simulink model "CompFeatures_eqHarness_req"  (R2012b)
settings: Solver=FixedStepDiscrete  StartTime=0.0  StopTime=50  RelTol=1e-3
InitFcn:
  | N=256;
  | Fs = 1000;
  | bw = 5.6;
undefined symbols (not defined in the file): sigbuilder_block
libraries: simulink x1
settings Model: RequirementInfo={'other' '..\..\..\requirements\ebd_srs.doc' '@Simulink_requirement_item_4' 'true' 'Filter input signal via polyphase digital filter bank' 'Requirement' } %GIDa_bfa4a348_cd9f_4101_a776_3ea215f34dae  SldvGeneratedHarnessModel=TestUnitModel=CompFeatures|  CovMetricSettings=dcmoe  CovHTMLOptions=-aTS=1 -bRG=1 -bTC=0 -hTR=0 -nFC=0 -scm=1 -bcm=1  CovModelRefEnable=on  CovExternalEMLEnable=on  Creator=aanantha  LastModifiedBy=klindqvi
settings DataIOCC: SaveFormat=StructureWithTime  SignalLoggingSaveFormat=ModelDataLogs  SaveOutput=off  SaveTime=off  SignalLoggingName=logsOut
settings OptimizationCC: InlineParams=on  OptimizeModelRefInitCode=on  LifeSpan=1
settings DebuggingCC: ReadBeforeWriteMsg=DisableAll  WriteAfterWriteMsg=DisableAll  WriteAfterReadMsg=DisableAll  InheritedTsInSrcMsg=none  ParameterPrecisionLossMsg=none  FcnCallInpInsideContextMsg=EnableAllAsWarning
settings HardwareCC: ProdLargestAtomicInteger=Long  ProdLargestAtomicFloat=Double  ProdEndianess=LittleEndian  ProdHWDeviceType=ARM Compatible->ARM Cortex
settings ModelReferenceCC: CheckModelReferenceTargetMessage=none
settings RTWCC: SystemTargetFile=ert.tlc  GenCodeOnly=on  TemplateMakefile=ert_default_tmf  Description=Embedded Coder  GenerateReport=on  ProcessScript=ert_make_rtw_hook  IncludeHyperlinkInReport=on  LaunchReport=on  GenerateTraceInfo=on  GenerateTraceReportSl=on  GenerateTraceReportSf=on  GenerateTraceReportEml=on  GenerateCodeMetricsReport=on
settings CodeAppCC: IgnoreCustomStorageClasses=off
settings ERTTargetCC: CodeReplacementLibrary=GCC ARM Cortex-A8  MultiwordLength=2048  GenerateSampleERTMain=on  ERTCustomFileTemplate=example_file_process.tlc  ConvertIfToSwitch=off  SuppressUnreachableDefaultCases=off

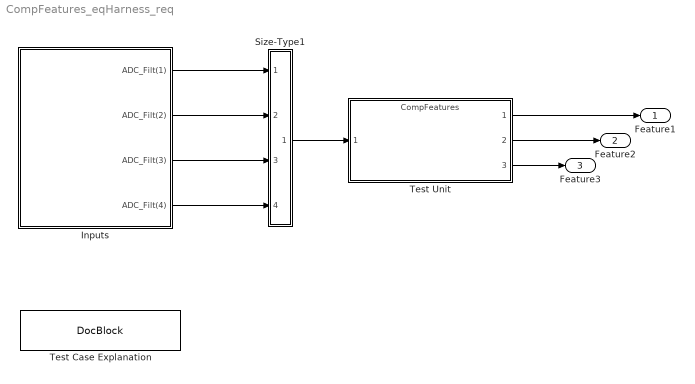
== system CompFeatures_eqHarness_req ==
  Inputs : Subsystem  Tag=STV Subsys  LoadFcn=sigbuilder_block('load',[49.5 50.25 519.75 603 ]);  StartFcn=sigbuilder_block('start');  StopFcn=sigbuilder_block('stop');  ClipboardFcn=sigbuilder_block('clipboard');  mask(Sigbuilder block){}
      mask init:
      | if ~strcmp(get_param(bdroot(gcb),'SimulationStatus'),'stopped'),tuvar = sigbuilder_block('maskInit'); end
      settings: CopyFcn=sigbuilder_block('copy');  DeleteFcn=sigbuilder_block('delete');  ModelCloseFcn=sigbuilder_block('modelClose');  PreSaveFcn=sigbuilder_block('preSave');  PauseFcn=sigbuilder_block('pause');  ContinueFcn=sigbuilder_block('continue');  NameChangeFcn=sigbuilder_block('namechange');  OpenFcn=sigbuilder_block('open',[49.5 50.25 519.75 603 ]);  CloseFcn=sigbuilder_block('close');
      mask Display: plot(0, 0, 100, 100,[2, 2, 32, 32, 2], [68, 8, 8, 68, 68],[32, 2], [38, 38], [32, 19, 2],[53, 60, 44], [32, 17, 17, 2],[16, 16, 31, 31]);txt = getActiveGroup(gcbh);text(2, 100, txt,'verticalAlignment', 'top');
  Size-Type1 : Subsystem
  Test Case Explanation : simulink/Model-Wide Utilities/DocBlock  DocumentType=Text
      content=|
      | Test case with default values because no SLDVDATA supplied
  Test Unit : ModelReference  ModelNameDialog=CompFeatures  SimulationMode=Normal  ModelReferenceVersion=1.277  CopyOfModelName=CompFeatures  DefaultDataLogging=on
  Feature1 : Outport  PortDimensions=1
  Feature2 : Outport  Port=2  PortDimensions=1  SampleTime=[0.08900000000000001,0]
  Feature3 : Outport  Port=3  PortDimensions=1  SampleTime=[0.08900000000000001,0]
  wires:
  Size-Type1/1(Out1) -> Test Unit/1
  Test Unit/1 -> Feature1/1
  Test Unit/2 -> Feature2/1
  Test Unit/3 -> Feature3/1
  Inputs/1(ADC_Filt(1)) -> Size-Type1/1(In1)
  Inputs/2(ADC_Filt(2)) -> Size-Type1/2(In2)
  Inputs/3(ADC_Filt(3)) -> Size-Type1/3(In3)
  Inputs/4(ADC_Filt(4)) -> Size-Type1/4(In4)

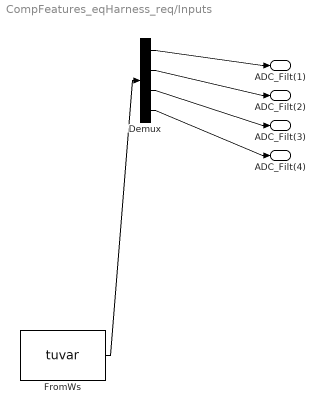
== system CompFeatures_eqHarness_req/Inputs ==
  Demux : Demux  Tag=STV Demux
  FromWs : FromWorkspace  Tag=STV FromWs  VariableName=tuvar  SampleTime=0
      SigBuilderData=|
      | dataSet(1).timeRange = [0 10]
      | dataSet(1).name = 'Test Case 1'
      | dataSet(2).timeRange = [0 10]
      | dataSet(2).name = 'Test Case 2'
      | sbobj.Name = 'Signal Builder'
      | sbobj.Groups(1).Name = 'Test Case 1'
      | sbobj.Groups(1).Signals(1).Name = 'ADC_Filt(1)'
      | sbobj.Groups(1).Signals(1).XData = [0 10]
      | sbobj.Groups(1).Signals(1).YData = [1 1]
      | sbobj.Groups(1).Signals(2).Name = 'ADC_Filt(2)'
      | sbobj.Groups(1).Signals(2).XData = [0 10]
      | sbobj.Groups(1).Signals(2).YData = [1 1]
      | sbobj.Groups(1).Signals(3).Name = 'ADC_Filt(3)'
      | sbobj.Groups(1).Signals(3).XData = [0 10]
      | sbobj.Groups(1).Signals(3).YData = [1 1]
      | sbobj.Groups(1).Signals(4).Name = 'ADC_Filt(4)'
      | sbobj.Groups(1).Signals(4).XData = [0 10]
      | sbobj.Groups(1).Signals(4).YData = [1 1]
      | sbobj.Groups(2).Name = 'Test Case 2'
      | sbobj.Groups(2).Signals(1).Name = 'ADC_Filt(1)'
      | sbobj.Groups(2).Signals(1).XData = [0 10]
      | sbobj.Groups(2).Signals(1).YData = [0 0]
      | sbobj.Groups(2).Signals(2).Name = 'ADC_Filt(2)'
      | sbobj.Groups(2).Signals(2).XData = [0 10]
      | sbobj.Groups(2).Signals(2).YData = [0 0]
      | sbobj.Groups(2).Signals(3).Name = 'ADC_Filt(3)'
      | sbobj.Groups(2).Signals(3).XData = [0 10]
      | sbobj.Groups(2).Signals(3).YData = [0 0]
      | sbobj.Groups(2).Signals(4).Name = 'ADC_Filt(4)'
      | sbobj.Groups(2).Signals(4).XData = [0 10]
      | sbobj.Groups(2).Signals(4).YData = [0 0]
  ADC_Filt(1) : Outport  Tag=STV Outport
  ADC_Filt(2) : Outport  Tag=STV Outport  Port=2
  ADC_Filt(3) : Outport  Tag=STV Outport  Port=3
  ADC_Filt(4) : Outport  Tag=STV Outport  Port=4
  wires:
  Demux/4 -> ADC_Filt(4)/1
  Demux/3 -> ADC_Filt(3)/1
  Demux/2 -> ADC_Filt(2)/1
  Demux/1 -> ADC_Filt(1)/1
  FromWs/1 -> Demux/1

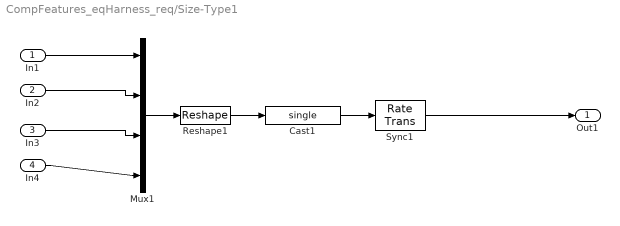
== system CompFeatures_eqHarness_req/Size-Type1 ==
  In1 : Inport
  In2 : Inport  Port=2
  In3 : Inport  Port=3
  In4 : Inport  Port=4
  Cast1 : DataTypeConversion  OutDataTypeStr=single  SaturateOnIntegerOverflow=on  RndMeth=Zero
  Mux1 : Mux
  Reshape1 : Reshape  OutputDimensionality=Customize  OutputDimensions=4
  Sync1 : RateTransition  OutPortSampleTime=[0.08900000000000001,0]
  Out1 : Outport
  wires:
  Sync1/1 -> Out1/1
  Cast1/1 -> Sync1/1
  Reshape1/1 -> Cast1/1
  Mux1/1 -> Reshape1/1
  In4/1 -> Mux1/4
  In3/1 -> Mux1/3
  In2/1 -> Mux1/2
  In1/1 -> Mux1/1
